simulink model "linuxTask"  (R2012b)
settings: Solver=FixedStepDiscrete  StartTime=0.0  StopTime=10.0  FixedStep=0.001  RelTol=1e-3
undefined symbols (not defined in the file): acquireMethods, autoplayMovementDuration, autoplayReactionTime, autoplayRotationDuration, autoplayRotationStart, centerOffset, clickPercentage, clickRefractoryPeriod, clickTargetColor, clickTargetHoverColor, cuedText, cuedTextLength, cumulativeDwell, cursorColorClick, cursorColorClosed, cursorColorOpen, cursorDiameter, cursorNeuralColor, cursorNonneuralColor, delayOrder, displayObject, dwellRefractoryPeriod, errorAssistAxis, errorAssistR, errorAssistTheta, expRandBinSize, expRandMax, expRandMin, expRandMu, failOnLiftoff, failurePenalty, falseClickFails, fingerPositionTolerance, fixedSeqMode, gain, gloveBias, gloveLPDenominator, gloveLPNumerator, gloveNonlinearCorrection, gloveXCorrection, gloveYCorrection, gridEdges, gridTilesEachDim, holdDuration, holdTime, initialInput, initialLockout, initialState, inputType, keyboard, keyboardDims, keyPressedTime, lockFingerPosition, maxTaskTime, memorizeMode, minTargetDistance, mouseLPDenominator, mouseLPNumerator, mouseOffset, movementDuration ... (+87)
settings Model: Creator=gilja  LastModifiedBy=NPTL
settings SolverCC: EnableConcurrentExecution=on  ConcurrentTasks=on
settings DataIOCC: SaveOutput=off  SignalLogging=off  SaveTime=off
settings OptimizationCC: InlineParams=on  InlineInvariantSignals=on  EnhancedBackFolding=on  EfficientFloat2IntCast=on  SimCompilerOptimization=On
settings DebuggingCC: UnderspecifiedInitializationDetection=Simplified
settings HardwareCC: ProdIntDivRoundTo=Zero  ProdEndianess=LittleEndian  ProdHWDeviceType=Generic->32-bit x86 compatible
settings ModelReferenceCC: ModelReferenceNumInstancesAllowed=Single  ModelReferenceMinAlgLoopOccurrences=on
settings RTWCC: SystemTargetFile=xpctarget.tlc  TemplateMakefile=xpc_default_tmf  Description=xPC Target  ProcessScript=xpctarget_make_rtw_hook  RTWCompilerOptimization=On
settings CodeAppCC: MaxIdLength=62
settings xpcTargetCC: TargetFcnLib=ansi_tfl_table_tmw.mat  CodeReplacementLibrary=XPC_BLAS  ParMdlRefBuildCompliant=on  ConcurrentExecutionCompliant=on  CombineSignalStateStructs=off  GRTInterface=on  xPCTaskExecutionProfile=on  xPCRL32EventNumber=5000  xPCisDownloadable=off  xPCLoadParamSetFile=off  xPCConcurrentTasks=off  xPCEnableSFAnimation=off

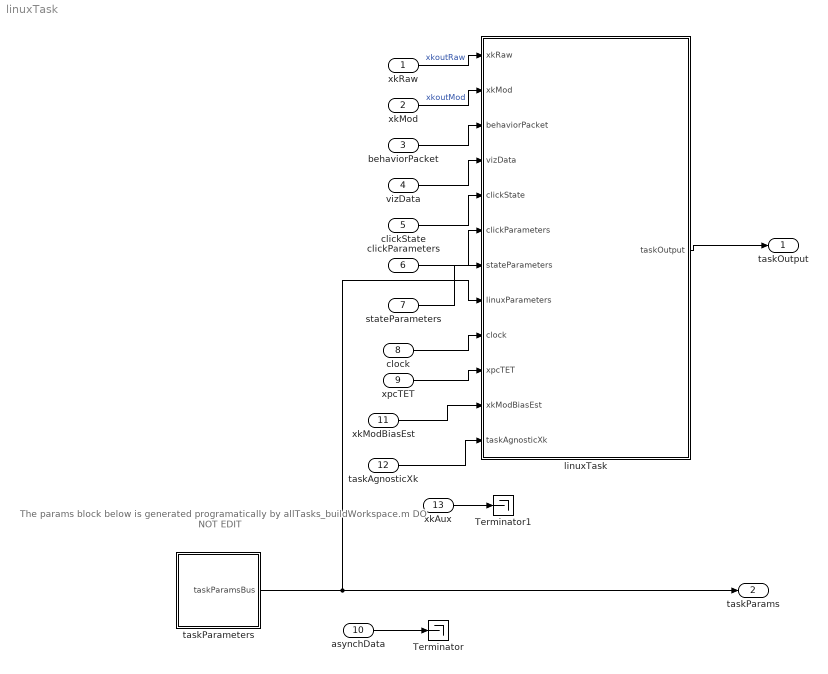
== system linuxTask ==
  note: The params block below is generated
      | programatically by allTasks_buildWorkspace.m
      | DO NOT EDIT
  xkRaw : Inport  OutDataTypeStr=double  PortDimensions=[double(xkConstants.NUM_STATE_DIMENSIONS),1]  SampleTime=[0.001,0]
  xkMod : Inport  Port=2  OutDataTypeStr=double  PortDimensions=[double(xkConstants.NUM_STATE_DIMENSIONS),1]  SampleTime=[0.001,0]
  behaviorPacket : Inport  Port=3  OutDataTypeStr=Bus: behaviorPacketBus  SampleTime=[0.001,0]
  vizData : Inport  Port=4  OutDataTypeStr=Bus: peripheralData  SampleTime=[0.001,0]
  clickState : Inport  Port=5  OutDataTypeStr=uint16  SampleTime=[0.001,0]
  clickParameters : Inport  Port=6  OutDataTypeStr=Bus: clickParametersBus  SampleTime=[0.001,0]
  stateParameters : Inport  Port=7  OutDataTypeStr=Bus: stateParams  SampleTime=[0.001,0]
  clock : Inport  Port=8  OutDataTypeStr=uint32  SampleTime=[0.001,0]
  xpcTET : Inport  Port=9  OutDataTypeStr=double  SampleTime=[0.001,0]
  asynchData : Inport  Port=10  OutDataTypeStr=Bus: peripheralData  SampleTime=[0.001,0]
  xkModBiasEst : Inport  Port=11  OutDataTypeStr=double  PortDimensions=[double(xkConstants.NUM_STATE_DIMENSIONS),1]  SampleTime=[0.001,0]
  taskAgnosticXk : Inport  Port=12  OutDataTypeStr=double  PortDimensions=[double(xkConstants.NUM_STATE_DIMENSIONS),1]  SampleTime=[0.001,0]
  xkAux : Inport  Port=13  OutDataTypeStr=double  PortDimensions=[double(xkConstants.NUM_STATE_DIMENSIONS),1]  SampleTime=[0.001,0]
  Terminator : Terminator
  Terminator1 : Terminator
  linuxTask : MATLAB Function  TreatAsAtomicUnit=on
  taskParameters : Subsystem
  taskOutput : Outport  OutDataTypeStr=Bus: taskOutput  SampleTime=[0.001,0]
  taskParams : Outport  Port=2  OutDataTypeStr=Bus: taskParamsBus  SampleTime=[0.001,0]
  wires:
  clickParameters/1 -> linuxTask/6(clickParameters)
  stateParameters/1 -> linuxTask/7(stateParameters)
  clock/1 -> linuxTask/9(clock)
  clickState/1 -> linuxTask/5(clickState)
  linuxTask/1(taskOutput) -> taskOutput/1
  xpcTET/1 -> linuxTask/10(xpcTET)
  vizData/1 -> linuxTask/4(vizData)
  behaviorPacket/1 -> linuxTask/3(behaviorPacket)
  asynchData/1 -> Terminator/1
  taskParameters/1(taskParamsBus) -> taskParams/1, linuxTask/8(linuxParameters)
  xkRaw/1 -> linuxTask/1(xkRaw)  "xkoutRaw"
  xkMod/1 -> linuxTask/2(xkMod)  "xkoutMod"
  xkModBiasEst/1 -> linuxTask/11(xkModBiasEst)
  taskAgnosticXk/1 -> linuxTask/12(taskAgnosticXk)
  xkAux/1 -> Terminator1/1

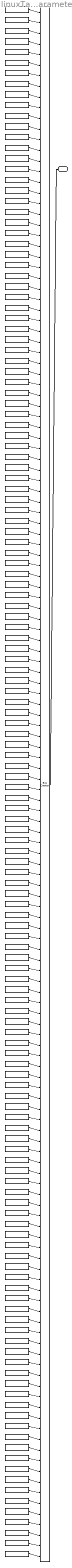
== system linuxTask/taskParameters ==
  BusOutput : BusCreator  Inputs=targetDiameter,maxTaskTime,holdTime,trialTimeout,numTrials,randomSeed,expRandMu,expRandMin,expRandMax,expRandBinSize,taskType,targetInds,numTargets,gain,failurePenalty,cursorDiameter,inputType,gloveBias,useRandomDelay,mouseOffset,workspaceX,workspaceY,workspaceZ,workspaceR,workspaceR2,showScores,trialsPerScore,cursorColorClick,recenterOnFail,recenterOnSuccess,recenterDelay,initialInput,clickPercentage,lockFingerPosition,fingerPositionTolerance,failOnLiftoff,errorAssistR,errorAssistTheta,errorAssistAxis,useGloveLPF,gloveLPNumerator,gloveLPDenominator,gloveNonlinearCorrection,gloveYCorrection,gloveXCorrection,useMouseLPF,soundOnFail,soundOnGo,soundOnSuccess,soundOnOverTarget,mouseLPNumerator,mouseLPDenominator,stopOffTarget,stopOnClick,outputType,xk2HorizontalPos,xk2HorizontalVel,xk2VerticalPos,xk2VerticalVel,xk2DepthPos,xk2DepthVel,xk2RotatePos,xk2RotateVel,xk2Rotate2Pos,xk2Rotate2Vel,gridEdges,gridTilesEachDim,selectionRefractoryMS,autoplayReactionTime,autoplayMovementDuration,powerGain,powerGainUnityCrossing,targetRotDiameter,autoplayRotationStart,autoplayRotationDuration,randomTaskTargetDiameters,randomTaskTargetRotDiameters,randomTaskBoundaries,numDisplayDims,cursorColorOpen,cursorColorClosed,showXYZaura,displayObject,preTrialLength,targetDiameters,numTargetDiameters,minTargetDistance,targetDelay,targetSpaceX,targetSpaceY,clickTargetColor,clickTargetHoverColor,falseClickFails,splitDimensions,vmrTheta,xkRawSpeedCap,movementDuration,holdDuration,restDuration,returnDuration,repsPerBlock,whichMovements,movementOrder,delayOrder,clickRefractoryPeriod,xpcVelocityOutputPeriodMS,outputVelocityScaling,screenUpdateRate,targetDevice,playSpokenCues,numTargetsInSeq,targetSeq,seqReadyTime,seqRehearseTime,rotateSeqCues,numRepsPerSeq,rehearsalOrder,rehearsalTimes,pathMode,memorizeMode,fixedSeqMode,sequenceMatrix,keyboard,resetDisplay,cursorNeuralColor,cursorNonneuralColor,centerOffset,scoreTime,cuedTextLength,cuedText,keyboardDims,recenterFullscreen,soundOnError,acquireMethods,cumulativeDwell,showBackspace,showStartStop,showTargetText,showTypedText,showCueOnTarget,showCueOffTarget,recenterOffset,dwellRefractoryPeriod,keyPressedTime,initialLockout,initialState  OutDataTypeStr=Bus: taskParamsBus
  acquireMethods : Constant  Value=acquireMethods
  autoplayMovementDuration : Constant  Value=autoplayMovementDuration
  autoplayReactionTime : Constant  Value=autoplayReactionTime
  autoplayRotationDuration : Constant  Value=autoplayRotationDuration
  autoplayRotationStart : Constant  Value=autoplayRotationStart
  centerOffset : Constant  Value=centerOffset
  clickPercentage : Constant  Value=clickPercentage
  clickRefractoryPeriod : Constant  Value=clickRefractoryPeriod
  clickTargetColor : Constant  Value=clickTargetColor
  clickTargetHoverColor : Constant  Value=clickTargetHoverColor
  cuedText : Constant  Value=cuedText
  cuedTextLength : Constant  Value=cuedTextLength
  cumulativeDwell : Constant  Value=cumulativeDwell
  cursorColorClick : Constant  Value=cursorColorClick
  cursorColorClosed : Constant  Value=cursorColorClosed
  cursorColorOpen : Constant  Value=cursorColorOpen
  cursorDiameter : Constant  Value=cursorDiameter
  cursorNeuralColor : Constant  Value=cursorNeuralColor
  cursorNonneuralColor : Constant  Value=cursorNonneuralColor
  delayOrder : Constant  Value=delayOrder
  displayObject : Constant  Value=displayObject
  dwellRefractoryPeriod : Constant  Value=dwellRefractoryPeriod
  errorAssistAxis : Constant  Value=errorAssistAxis
  errorAssistR : Constant  Value=errorAssistR
  errorAssistTheta : Constant  Value=errorAssistTheta
  expRandBinSize : Constant  Value=expRandBinSize
  expRandMax : Constant  Value=expRandMax
  expRandMin : Constant  Value=expRandMin
  expRandMu : Constant  Value=expRandMu
  failOnLiftoff : Constant  Value=failOnLiftoff
  failurePenalty : Constant  Value=failurePenalty
  falseClickFails : Constant  Value=falseClickFails
  fingerPositionTolerance : Constant  Value=fingerPositionTolerance
  fixedSeqMode : Constant  Value=fixedSeqMode
  gain : Constant  Value=gain
  gloveBias : Constant  Value=gloveBias
  gloveLPDenominator : Constant  Value=gloveLPDenominator
  gloveLPNumerator : Constant  Value=gloveLPNumerator
  gloveNonlinearCorrection : Constant  Value=gloveNonlinearCorrection
  gloveXCorrection : Constant  Value=gloveXCorrection
  gloveYCorrection : Constant  Value=gloveYCorrection
  gridEdges : Constant  Value=gridEdges
  gridTilesEachDim : Constant  Value=gridTilesEachDim
  holdDuration : Constant  Value=holdDuration
  holdTime : Constant  Value=holdTime
  initialInput : Constant  Value=initialInput
  initialLockout : Constant  Value=initialLockout
  initialState : Constant  Value=initialState
  inputType : Constant  Value=inputType
  keyPressedTime : Constant  Value=keyPressedTime
  keyboard : Constant  Value=keyboard
  keyboardDims : Constant  Value=keyboardDims
  lockFingerPosition : Constant  Value=lockFingerPosition
  maxTaskTime : Constant  Value=maxTaskTime
  memorizeMode : Constant  Value=memorizeMode
  minTargetDistance : Constant  Value=minTargetDistance
  mouseLPDenominator : Constant  Value=mouseLPDenominator
  mouseLPNumerator : Constant  Value=mouseLPNumerator
  mouseOffset : Constant  Value=mouseOffset
  movementDuration : Constant  Value=movementDuration
  movementOrder : Constant  Value=movementOrder
  numDisplayDims : Constant  Value=numDisplayDims
  numRepsPerSeq : Constant  Value=numRepsPerSeq
  numTargetDiameters : Constant  Value=numTargetDiameters
  numTargets : Constant  Value=numTargets
  numTargetsInSeq : Constant  Value=numTargetsInSeq
  numTrials : Constant  Value=numTrials
  outputType : Constant  Value=outputType
  outputVelocityScaling : Constant  Value=outputVelocityScaling
  pathMode : Constant  Value=pathMode
  playSpokenCues : Constant  Value=playSpokenCues
  powerGain : Constant  Value=powerGain
  powerGainUnityCrossing : Constant  Value=powerGainUnityCrossing
  preTrialLength : Constant  Value=preTrialLength
  randomSeed : Constant  Value=randomSeed
  randomTaskBoundaries : Constant  Value=randomTaskBoundaries
  randomTaskTargetDiameters : Constant  Value=randomTaskTargetDiameters
  randomTaskTargetRotDiameters : Constant  Value=randomTaskTargetRotDiameters
  recenterDelay : Constant  Value=recenterDelay
  recenterFullscreen : Constant  Value=recenterFullscreen
  recenterOffset : Constant  Value=recenterOffset
  recenterOnFail : Constant  Value=recenterOnFail
  recenterOnSuccess : Constant  Value=recenterOnSuccess
  rehearsalOrder : Constant  Value=rehearsalOrder
  rehearsalTimes : Constant  Value=rehearsalTimes
  repsPerBlock : Constant  Value=repsPerBlock
  resetDisplay : Constant  Value=resetDisplay
  restDuration : Constant  Value=restDuration
  returnDuration : Constant  Value=returnDuration
  rotateSeqCues : Constant  Value=rotateSeqCues
  scoreTime : Constant  Value=scoreTime
  screenUpdateRate : Constant  Value=screenUpdateRate
  selectionRefractoryMS : Constant  Value=selectionRefractoryMS
  seqReadyTime : Constant  Value=seqReadyTime
  seqRehearseTime : Constant  Value=seqRehearseTime
  sequenceMatrix : Constant  Value=sequenceMatrix
  showBackspace : Constant  Value=showBackspace
  showCueOffTarget : Constant  Value=showCueOffTarget
  showCueOnTarget : Constant  Value=showCueOnTarget
  showScores : Constant  Value=showScores
  showStartStop : Constant  Value=showStartStop
  showTargetText : Constant  Value=showTargetText
  showTypedText : Constant  Value=showTypedText
  showXYZaura : Constant  Value=showXYZaura
  soundOnError : Constant  Value=soundOnError
  soundOnFail : Constant  Value=soundOnFail
  soundOnGo : Constant  Value=soundOnGo
  soundOnOverTarget : Constant  Value=soundOnOverTarget
  soundOnSuccess : Constant  Value=soundOnSuccess
  splitDimensions : Constant  Value=splitDimensions
  stopOffTarget : Constant  Value=stopOffTarget
  stopOnClick : Constant  Value=stopOnClick
  targetDelay : Constant  Value=targetDelay
  targetDevice : Constant  Value=targetDevice
  targetDiameter : Constant  Value=targetDiameter
  targetDiameters : Constant  Value=targetDiameters
  targetInds : Constant  Value=targetInds
  targetRotDiameter : Constant  Value=targetRotDiameter
  targetSeq : Constant  Value=targetSeq
  targetSpaceX : Constant  Value=targetSpaceX
  targetSpaceY : Constant  Value=targetSpaceY
  taskType : Constant  Value=taskType
  trialTimeout : Constant  Value=trialTimeout
  trialsPerScore : Constant  Value=trialsPerScore
  useGloveLPF : Constant  Value=useGloveLPF
  useMouseLPF : Constant  Value=useMouseLPF
  useRandomDelay : Constant  Value=useRandomDelay
  vmrTheta : Constant  Value=vmrTheta
  whichMovements : Constant  Value=whichMovements
  workspaceR : Constant  Value=workspaceR
  workspaceR2 : Constant  Value=workspaceR2
  workspaceX : Constant  Value=workspaceX
  workspaceY : Constant  Value=workspaceY
  workspaceZ : Constant  Value=workspaceZ
  xk2DepthPos : Constant  Value=xk2DepthPos
  xk2DepthVel : Constant  Value=xk2DepthVel
  xk2HorizontalPos : Constant  Value=xk2HorizontalPos
  xk2HorizontalVel : Constant  Value=xk2HorizontalVel
  xk2Rotate2Pos : Constant  Value=xk2Rotate2Pos
  xk2Rotate2Vel : Constant  Value=xk2Rotate2Vel
  xk2RotatePos : Constant  Value=xk2RotatePos
  xk2RotateVel : Constant  Value=xk2RotateVel
  xk2VerticalPos : Constant  Value=xk2VerticalPos
  xk2VerticalVel : Constant  Value=xk2VerticalVel
  xkRawSpeedCap : Constant  Value=xkRawSpeedCap
  xpcVelocityOutputPeriodMS : Constant  Value=xpcVelocityOutputPeriodMS
  taskParamsBus : Outport
  wires:
  targetDiameter/1 -> BusOutput/1  "targetDiameter"
  maxTaskTime/1 -> BusOutput/2  "maxTaskTime"
  holdTime/1 -> BusOutput/3  "holdTime"
  trialTimeout/1 -> BusOutput/4  "trialTimeout"
  numTrials/1 -> BusOutput/5  "numTrials"
  randomSeed/1 -> BusOutput/6  "randomSeed"
  expRandMu/1 -> BusOutput/7  "expRandMu"
  expRandMin/1 -> BusOutput/8  "expRandMin"
  expRandMax/1 -> BusOutput/9  "expRandMax"
  expRandBinSize/1 -> BusOutput/10  "expRandBinSize"
  taskType/1 -> BusOutput/11  "taskType"
  targetInds/1 -> BusOutput/12  "targetInds"
  numTargets/1 -> BusOutput/13  "numTargets"
  gain/1 -> BusOutput/14  "gain"
  failurePenalty/1 -> BusOutput/15  "failurePenalty"
  cursorDiameter/1 -> BusOutput/16  "cursorDiameter"
  inputType/1 -> BusOutput/17  "inputType"
  gloveBias/1 -> BusOutput/18  "gloveBias"
  useRandomDelay/1 -> BusOutput/19  "useRandomDelay"
  mouseOffset/1 -> BusOutput/20  "mouseOffset"
  workspaceX/1 -> BusOutput/21  "workspaceX"
  workspaceY/1 -> BusOutput/22  "workspaceY"
  workspaceZ/1 -> BusOutput/23  "workspaceZ"
  workspaceR/1 -> BusOutput/24  "workspaceR"
  workspaceR2/1 -> BusOutput/25  "workspaceR2"
  showScores/1 -> BusOutput/26  "showScores"
  trialsPerScore/1 -> BusOutput/27  "trialsPerScore"
  cursorColorClick/1 -> BusOutput/28  "cursorColorClick"
  recenterOnFail/1 -> BusOutput/29  "recenterOnFail"
  recenterOnSuccess/1 -> BusOutput/30  "recenterOnSuccess"
  recenterDelay/1 -> BusOutput/31  "recenterDelay"
  initialInput/1 -> BusOutput/32  "initialInput"
  clickPercentage/1 -> BusOutput/33  "clickPercentage"
  lockFingerPosition/1 -> BusOutput/34  "lockFingerPosition"
  fingerPositionTolerance/1 -> BusOutput/35  "fingerPositionTolerance"
  failOnLiftoff/1 -> BusOutput/36  "failOnLiftoff"
  errorAssistR/1 -> BusOutput/37  "errorAssistR"
  errorAssistTheta/1 -> BusOutput/38  "errorAssistTheta"
  errorAssistAxis/1 -> BusOutput/39  "errorAssistAxis"
  useGloveLPF/1 -> BusOutput/40  "useGloveLPF"
  gloveLPNumerator/1 -> BusOutput/41  "gloveLPNumerator"
  gloveLPDenominator/1 -> BusOutput/42  "gloveLPDenominator"
  gloveNonlinearCorrection/1 -> BusOutput/43  "gloveNonlinearCorrection"
  gloveYCorrection/1 -> BusOutput/44  "gloveYCorrection"
  gloveXCorrection/1 -> BusOutput/45  "gloveXCorrection"
  useMouseLPF/1 -> BusOutput/46  "useMouseLPF"
  soundOnFail/1 -> BusOutput/47  "soundOnFail"
  soundOnGo/1 -> BusOutput/48  "soundOnGo"
  soundOnSuccess/1 -> BusOutput/49  "soundOnSuccess"
  soundOnOverTarget/1 -> BusOutput/50  "soundOnOverTarget"
  mouseLPNumerator/1 -> BusOutput/51  "mouseLPNumerator"
  mouseLPDenominator/1 -> BusOutput/52  "mouseLPDenominator"
  stopOffTarget/1 -> BusOutput/53  "stopOffTarget"
  stopOnClick/1 -> BusOutput/54  "stopOnClick"
  outputType/1 -> BusOutput/55  "outputType"
  xk2HorizontalPos/1 -> BusOutput/56  "xk2HorizontalPos"
  xk2HorizontalVel/1 -> BusOutput/57  "xk2HorizontalVel"
  xk2VerticalPos/1 -> BusOutput/58  "xk2VerticalPos"
  xk2VerticalVel/1 -> BusOutput/59  "xk2VerticalVel"
  xk2DepthPos/1 -> BusOutput/60  "xk2DepthPos"
  xk2DepthVel/1 -> BusOutput/61  "xk2DepthVel"
  xk2RotatePos/1 -> BusOutput/62  "xk2RotatePos"
  xk2RotateVel/1 -> BusOutput/63  "xk2RotateVel"
  xk2Rotate2Pos/1 -> BusOutput/64  "xk2Rotate2Pos"
  xk2Rotate2Vel/1 -> BusOutput/65  "xk2Rotate2Vel"
  gridEdges/1 -> BusOutput/66  "gridEdges"
  gridTilesEachDim/1 -> BusOutput/67  "gridTilesEachDim"
  selectionRefractoryMS/1 -> BusOutput/68  "selectionRefractoryMS"
  autoplayReactionTime/1 -> BusOutput/69  "autoplayReactionTime"
  autoplayMovementDuration/1 -> BusOutput/70  "autoplayMovementDuration"
  powerGain/1 -> BusOutput/71  "powerGain"
  powerGainUnityCrossing/1 -> BusOutput/72  "powerGainUnityCrossing"
  targetRotDiameter/1 -> BusOutput/73  "targetRotDiameter"
  autoplayRotationStart/1 -> BusOutput/74  "autoplayRotationStart"
  autoplayRotationDuration/1 -> BusOutput/75  "autoplayRotationDuration"
  randomTaskTargetDiameters/1 -> BusOutput/76  "randomTaskTargetDiameters"
  randomTaskTargetRotDiameters/1 -> BusOutput/77  "randomTaskTargetRotDiameters"
  randomTaskBoundaries/1 -> BusOutput/78  "randomTaskBoundaries"
  numDisplayDims/1 -> BusOutput/79  "numDisplayDims"
  cursorColorOpen/1 -> BusOutput/80  "cursorColorOpen"
  cursorColorClosed/1 -> BusOutput/81  "cursorColorClosed"
  showXYZaura/1 -> BusOutput/82  "showXYZaura"
  displayObject/1 -> BusOutput/83  "displayObject"
  preTrialLength/1 -> BusOutput/84  "preTrialLength"
  targetDiameters/1 -> BusOutput/85  "targetDiameters"
  numTargetDiameters/1 -> BusOutput/86  "numTargetDiameters"
  minTargetDistance/1 -> BusOutput/87  "minTargetDistance"
  targetDelay/1 -> BusOutput/88  "targetDelay"
  targetSpaceX/1 -> BusOutput/89  "targetSpaceX"
  targetSpaceY/1 -> BusOutput/90  "targetSpaceY"
  clickTargetColor/1 -> BusOutput/91  "clickTargetColor"
  clickTargetHoverColor/1 -> BusOutput/92  "clickTargetHoverColor"
  falseClickFails/1 -> BusOutput/93  "falseClickFails"
  splitDimensions/1 -> BusOutput/94  "splitDimensions"
  vmrTheta/1 -> BusOutput/95  "vmrTheta"
  xkRawSpeedCap/1 -> BusOutput/96  "xkRawSpeedCap"
  movementDuration/1 -> BusOutput/97  "movementDuration"
  holdDuration/1 -> BusOutput/98  "holdDuration"
  restDuration/1 -> BusOutput/99  "restDuration"
  returnDuration/1 -> BusOutput/100  "returnDuration"
  repsPerBlock/1 -> BusOutput/101  "repsPerBlock"
  whichMovements/1 -> BusOutput/102  "whichMovements"
  movementOrder/1 -> BusOutput/103  "movementOrder"
  delayOrder/1 -> BusOutput/104  "delayOrder"
  clickRefractoryPeriod/1 -> BusOutput/105  "clickRefractoryPeriod"
  xpcVelocityOutputPeriodMS/1 -> BusOutput/106  "xpcVelocityOutputPeriodMS"
  outputVelocityScaling/1 -> BusOutput/107  "outputVelocityScaling"
  screenUpdateRate/1 -> BusOutput/108  "screenUpdateRate"
  targetDevice/1 -> BusOutput/109  "targetDevice"
  playSpokenCues/1 -> BusOutput/110  "playSpokenCues"
  numTargetsInSeq/1 -> BusOutput/111  "numTargetsInSeq"
  targetSeq/1 -> BusOutput/112  "targetSeq"
  seqReadyTime/1 -> BusOutput/113  "seqReadyTime"
  seqRehearseTime/1 -> BusOutput/114  "seqRehearseTime"
  rotateSeqCues/1 -> BusOutput/115  "rotateSeqCues"
  numRepsPerSeq/1 -> BusOutput/116  "numRepsPerSeq"
  rehearsalOrder/1 -> BusOutput/117  "rehearsalOrder"
  rehearsalTimes/1 -> BusOutput/118  "rehearsalTimes"
  pathMode/1 -> BusOutput/119  "pathMode"
  memorizeMode/1 -> BusOutput/120  "memorizeMode"
  fixedSeqMode/1 -> BusOutput/121  "fixedSeqMode"
  sequenceMatrix/1 -> BusOutput/122  "sequenceMatrix"
  keyboard/1 -> BusOutput/123  "keyboard"
  resetDisplay/1 -> BusOutput/124  "resetDisplay"
  cursorNeuralColor/1 -> BusOutput/125  "cursorNeuralColor"
  cursorNonneuralColor/1 -> BusOutput/126  "cursorNonneuralColor"
  centerOffset/1 -> BusOutput/127  "centerOffset"
  scoreTime/1 -> BusOutput/128  "scoreTime"
  cuedTextLength/1 -> BusOutput/129  "cuedTextLength"
  cuedText/1 -> BusOutput/130  "cuedText"
  keyboardDims/1 -> BusOutput/131  "keyboardDims"
  recenterFullscreen/1 -> BusOutput/132  "recenterFullscreen"
  soundOnError/1 -> BusOutput/133  "soundOnError"
  acquireMethods/1 -> BusOutput/134  "acquireMethods"
  cumulativeDwell/1 -> BusOutput/135  "cumulativeDwell"
  showBackspace/1 -> BusOutput/136  "showBackspace"
  showStartStop/1 -> BusOutput/137  "showStartStop"
  showTargetText/1 -> BusOutput/138  "showTargetText"
  showTypedText/1 -> BusOutput/139  "showTypedText"
  showCueOnTarget/1 -> BusOutput/140  "showCueOnTarget"
  showCueOffTarget/1 -> BusOutput/141  "showCueOffTarget"
  recenterOffset/1 -> BusOutput/142  "recenterOffset"
  dwellRefractoryPeriod/1 -> BusOutput/143  "dwellRefractoryPeriod"
  keyPressedTime/1 -> BusOutput/144  "keyPressedTime"
  initialLockout/1 -> BusOutput/145  "initialLockout"
  initialState/1 -> BusOutput/146  "initialState"
  BusOutput/1 -> taskParamsBus/1

== matlab function linuxTask/linuxTask ==
  data: xkRaw input double size=[double(xkConstants.NUM_STATE_DIMENSIONS) 1]; xkMod input; behaviorPacket input Bus: behaviorPacketBus size=1; vizData input Bus: peripheralData; clickState input; clickParameters input; taskOutput output Bus: taskOutput; stateParameters input Bus: stateParams size=1; linuxParameters input Bus: taskParamsBus; clock input; xpcTET input; xkModBiasEst input; taskAgnosticXk input
function taskOutput  = linuxTask(xkRaw, xkMod, behaviorPacket, vizData, clickState, clickParameters, stateParameters, linuxParameters, clock, xpcTET, xkModBiasEst, taskAgnosticXk)
%#codegen

mouse = behaviorPacket.mouse(1:6);
glove = behaviorPacket.glove(1:5);
behaviorRequestClock = behaviorPacket.xpcRequestClock;
peripheralTimestamp = behaviorPacket.peripheralTimestamp(1:16);

%% CONSTANTS
TASK_NAME = 'linux';
VERSION_ID = single(2.001);  % Changed August 23 2016; BJ: updated to 2.001 with splitting of xk into xkRaw and xkMod.
NUM_DIMS = uint8(cursorConstants.NUM_DIMENSIONS); % dimensionality of the task. August 2016 raised this from 2 to 3
STATEVEC_SIZE = double( xkConstants.NUM_STATE_DIMENSIONS ); % SDS July 2016
INIT_TIME = uint32(2000);


%% INITIALIZE TASK OUTPUT
fileLoggerData.data = uint8(zeros(1,1400));
fileLoggerData.dataLen = uint16(0);
fileLoggerData.fileName = uint8(zeros(1,20));
fileLoggerData.send = false;

fileLoggerFormat.format = uint8(zeros(1,1400));
fileLoggerFormat.formatLen = uint16(0);
fileLoggerFormat.fileName = uint8(zeros(1,20));

fileLoggerFormatAndData.format = fileLoggerFormat;
fileLoggerFormatAndData.data = fileLoggerData;

taskOutput.flushFiles = false;
taskOutput.sendFormat = false;
taskOutput.taskDetails = fileLoggerFormat;
taskOutput.discrete = fileLoggerFormatAndData;
taskOutput.continuous = fileLoggerFormatAndData;
taskOutput.screen = fileLoggerFormatAndData;
taskOutput.sound = fileLoggerFormatAndData;
taskOutput.asynch = fileLoggerFormatAndData;
taskOutput.ttl = double(0);
taskOutput.xk = xkRaw;
taskOutput.inputType = linuxParameters.initialInput;
taskOutput.currentTarget = single(zeros([double(xkConstants.NUM_TARGET_DIMENSIONS) 1]));
taskOutput.state = uint16(0);
taskOutput.paused = false;
taskOutput.allowStop = true;
taskOutput.resetHMM = false;

% taskOutput.flushFiles = false;
% taskOutput.sendFormat = false;
% taskOutput.taskDetails = fileLoggerFormat;
% taskOutput.discrete = fileLoggerFormatAndData;
% taskOutput.continuous = fileLoggerFormatAndData;
% taskOutput.screen = fileLoggerFormatAndData;
% taskOutput.sound = fileLoggerFormatAndData;
% taskOutput.xk = xk;
% taskOutput.inputType = linuxParameters.initialInput;

%% TASK DETAILS PACKET
taskOutput.taskDetails = packFileLoggerTaskDetails(TASK_NAME, VERSION_ID, ...
    'STATE_INIT', uint32(LinuxStates.STATE_INIT), ...
    'STATE_FREE_RUN', uint32(LinuxStates.STATE_FREE_RUN),...
    'STATE_PAUSE', uint32(LinuxStates.STATE_PAUSE),...
    'STATE_END', uint32(LinuxStates.STATE_END),...
    'TASK_CENTER_OUT', uint32(linuxConstants.TASK_FREE_RUN), ...
    'NUM_DIMENSIONS', uint32(DecoderConstants.NUM_KINEMATIC_DIMENSIONS), ...
    'INPUT_TYPE_MOUSE_ABSOLUTE', uint8(cursorConstants.INPUT_TYPE_MOUSE_ABSOLUTE), ...
    'INPUT_TYPE_DECODE_V', uint8(cursorConstants.INPUT_TYPE_DECODE_V)...
);



%% DEFINE PERSISTENTS
persistent state vizPacket;
persistent pauseTriggered;
persistent stateTimer;

persistent lockedParameters inputType;

persistent lastSoundTime;
persistent lastSoundState;

persistent clickTimer;
persistent lastClickTime;
persistent lastClickState;

persistent latchedXk;

%%initialize local vars
clickStateOut = uint16(0);

%% INITIALIZE PERSISTENTS
if(isempty(state))
    state = uint16(LinuxStates.STATE_INIT);
    
    vizPacket = initVizPacket;
    stateTimer = uint16(0);
    pauseTriggered = true;
    
    %BJ: xk was initialized here as follows; I'm replacing xk with xkMod and initializing xkRaw to the same thing: 
    xkMod = double(zeros([STATEVEC_SIZE 1]));
    xkMod(end,1) = 1;
    xkRaw = xkMod;
    
    %% buffer all the parameters off the bus
    lockedParameters = linuxParameters;
    inputType = lockedParameters.initialInput;
    
    lastSoundTime = clock;
    lastSoundState = uint8(LinuxStates.SOUND_STATE_IDLE);

    clickTimer = uint16(0);
    lastClickState = uint16(0);
    lastClickTime = uint32(0);
    latchedXk = xkMod;
end

%% update parameters on every cycle
lockedParameters = linuxParameters;
inputType = lockedParameters.inputType;

%% which state elements do I look to for the cursor's position? SDS August 2016
xk2HorizontalPos = uint8( lockedParameters.xk2HorizontalPos );
xk2VerticalPos = uint8( lockedParameters.xk2VerticalPos );
xk2HorizontalVel = uint8( lockedParameters.xk2HorizontalVel );
xk2VerticalVel = uint8( lockedParameters.xk2VerticalVel );
effectorPosInds = [xk2HorizontalPos, xk2VerticalPos];
effectorVelInds = [xk2HorizontalVel, xk2VerticalVel];

if clickState == uint16(DiscreteStates.CLICK_MAIN)
    clickTimer = clickTimer+uint16(1);
else
    clickTimer = uint16(0);
end

if uint32(clock-lastClickTime) < uint32(lockedParameters.clickRefractoryPeriod)
    clickTimer = uint16(0);
end


if(clock < INIT_TIME)
    pauseTriggered = true;
end

% We usually shouldn't write discrete data
writeDiscreteData = false;

if(vizData.receive && (vizData.dataLen > 0 ))
    vizPacket = parseVizPacket(vizData.data);
end



    %% STATE MACHINE
    switch state
        case {LinuxStates.STATE_INIT}
            %% set all the persistents that may have been changed by user input
            pauseTriggered = stateParameters.pause;
            stateTimer = stateTimer + 1;
            clickStateOut = uint16(0);
            if ~pauseTriggered
                stateTimer = uint16(0);
                state = uint16(LinuxStates.STATE_FREE_RUN);
                writeDiscreteData = true; %send out a discrete packet on state toggles
            end
            
        case {LinuxStates.STATE_FREE_RUN}
            stateTimer = stateTimer + 1;
            pauseTriggered = stateParameters.pause;
            if (clickTimer > clickParameters.clickHoldTime)
                clickStateOut = uint16(DiscreteStates.CLICK_MAIN);
            else
                clickStateOut = uint16(0);
            end
            
            if (clickStateOut && clickStateOut ~=lastClickState)
                lastClickTime = clock;
                lastSoundTime = clock;
                lastSoundState = uint8(LinuxStates.SOUND_STATE_CLICK);
            end
            if pauseTriggered
                stateTimer = uint16(0);
                state = uint16(LinuxStates.STATE_PAUSE);
            end
            
        case {LinuxStates.STATE_PAUSE}
            pauseTriggered = stateParameters.pause;
            stateTimer = stateTimer + 1;
            clickStateOut = uint16(0);
            if ~pauseTriggered
                stateTimer = uint16(0);
                state = uint16(LinuxStates.STATE_FREE_RUN);
            end
            
%% don't know how we would ever get here.            
        case {LinuxStates.STATE_END}
            stateTimer = stateTimer + 1;
            
    end

taskOutput.xk = xkRaw;  %BJ: this was already initialized above, in INITIALIZE TASK OUTPUT; here again in case state was empty, perhaps?
taskOutput.state = uint16(state);

%% latch the output to the visualization system
if lockedParameters.xpcVelocityOutputPeriodMS <= 1
    latchedXk = xkMod;
    sendVizData = true;
else
    if mod(double(clock), double(lockedParameters.xpcVelocityOutputPeriodMS)) == 0
        latchedXk(effectorPosInds) = xkMod(effectorPosInds);
        latchedXk(effectorVelInds) = latchedXk(effectorVelInds) + xkMod(effectorVelInds);
%         latchedXk(end) = xk(end); %1 term, I don't think this is necessary
        sendVizData = true;
    elseif mod(double(clock), double(lockedParameters.xpcVelocityOutputPeriodMS)) == 1
        latchedXk = xkMod;
        sendVizData = false;
    else
        latchedXk(effectorPosInds) = xkMod(effectorPosInds);
        latchedXk(effectorVelInds) = latchedXk(effectorVelInds) + xkMod(effectorVelInds);
%         latchedXk(5) = xk(5);        
        sendVizData = false;
    end
end
% latchedXk = xkMod; %xkRaw; % TEMP HACK TO DEBUG SDS JAN 9 2018

taskOutput.screen.data.send = sendVizData;

taskAgnosticVel = single(taskAgnosticXk(effectorVelInds)');

%% PACK DATA FOR CONTINUOUS OUTPUT
taskOutput.continuous = packFileLoggerFormatAndData('continuous', ...
    TASK_NAME, VERSION_ID, ...
    'clock', clock, ...
    'pause', pauseTriggered, ...
    'xpcRequestClock', behaviorRequestClock, ...
    'peripheralTimestamp', peripheralTimestamp, ...
    'state', state, ...
    'inputType', inputType, ...
    'mouse', mouse, ...
    'glove', glove, ...
    'clickState', uint16(clickStateOut), ...
    'clickTimer', clickTimer, ...
    'xpcScreenUpdateClock',vizPacket.xpcScreenUpdateClock,...
    'outputVelocityScaling',lockedParameters.outputVelocityScaling,...
    'sendVizData', sendVizData,...
    'cursorPosition', single(xkMod(effectorPosInds)), ...
    'xk', single(taskOutput.xk),...
    'cursorPosition',  latchedXk(effectorPosInds),...
    'cursorVelocity', latchedXk(effectorVelInds),...
    'stateTimer', stateTimer, ...
    'xpcTET', single(xpcTET), ...
    'xkModBiasEst', single(xkModBiasEst), ...
    'taskAgnosticVel', taskAgnosticVel(1:NUM_DIMS) ...
    );

%% SEND DISCRETE DATA TO FILELOGGER
taskOutput.discrete = packFileLoggerFormatAndData('discrete', ...
    TASK_NAME, VERSION_ID, ...
    'clock', clock,...
    'state', state, ...
    'taskType', lockedParameters.taskType, ...
    'gain', lockedParameters.gain, ...
    'mouseOffset', lockedParameters.mouseOffset, ...
    'screenUpdateRate',lockedParameters.screenUpdateRate,...
    'targetDevice',lockedParameters.targetDevice,...
    'xpcVelocityOutputPeriodMS',lockedParameters.xpcVelocityOutputPeriodMS,...
    'inputType', inputType, ...
    'useGloveLPF', uint8(lockedParameters.useGloveLPF),...
    'hmmClickSpeedMax',single(clickParameters.hmmClickSpeedMax),...
    'outputVelocityScaling',lockedParameters.outputVelocityScaling,...
    'workspaceX', lockedParameters.workspaceX, ...
    'workspacey', lockedParameters.workspaceY ...
    );

    
%% SEND DATA OUT TO VIZ
taskOutput.screen = packFileLoggerFormatAndData('screen', ...
    TASK_NAME, VERSION_ID, ...
    'clock', clock,...
    'state',state,...
    'cursorPosition',  latchedXk(effectorPosInds),...
    'cursorVelocity', latchedXk(effectorVelInds),...
    'targetDevice', lockedParameters.targetDevice, ...
    'screenUpdateRate',lockedParameters.screenUpdateRate,...
    'outputVelocityScaling',lockedParameters.outputVelocityScaling,...
    'clickState', uint16(clickStateOut), ...
    'inputType', inputType,...
    'taskType', lockedParameters.taskType...
    ); 

%% SEND DATA OUT TO SOUND
taskOutput.sound = packFileLoggerFormatAndData('screen', ...
    TASK_NAME, VERSION_ID, ...
    'clock', clock,...
    'vizState',state,...
    'lastSoundTime',lastSoundTime,...
    'lastSoundState',lastSoundState...
    ); 


%% SET SEND FLAGS FOR NETWORK OUTPUTS
if(clock < INIT_TIME)
    taskOutput.discrete.data.send = false;
    taskOutput.continuous.data.send = false;
    taskOutput.screen.data.send = false;
    taskOutput.sound.data.send = false;
    
    if(mod(clock, 10)==0)
        taskOutput.sendFormat = true;
    else
        taskOutput.sendFormat = false;
    end
    stateTimer = uint16(0);
else
    taskOutput.discrete.data.send = writeDiscreteData;
    taskOutput.continuous.data.send = true;
    taskOutput.screen.data.send = sendVizData;
    taskOutput.sound.data.send = true;
    taskOutput.sendFormat = false;
    taskOutput.inputType = inputType;
end

taskOutput.paused = pauseTriggered;
lastState = state;

end



function vizPacket = parseVizPacket(packetData)

    vizPacket.xpcScreenUpdateClock = typecast(packetData(28+[1:4]), 'uint32');

end

function vizPacket = initVizPacket()

    vizPacket.xpcScreenUpdateClock = uint32(0);

end
